simulink model "Tarea1"  (R2022a)
settings: Solver=VariableStepAuto  StartTime=0.0  StopTime=10.0  RelTol=1e-3
values from neighbouring files (symbols this model uses):
  den = [0 (L*J) (R*J+L*B) (R*B+Km*Ka)]    [CompensadordicretoVelocidadLGR.m]    (also in Grafica_FuncionDeTransferencia.m = [1 0,1486 0,04365]; PIDExperiment.m = str2num(get(handles.den,'string')); Raices.m = [1 12.02 0.1393]; Smulacro_Parcial_Final.m = [1 0 30 15])
  num = [0 (Km)]    [CompensadordicretoVelocidadLGR.m]    (also in Grafica_FuncionDeTransferencia.m = [0,2087 0,1993]; PIDExperiment.m = str2num(get(handles.num,'string')); Raices.m = [0.393 0.2155]; Smulacro_Parcial_Final.m = [1 2])
settings Model: Creator=juane  LastModifiedBy=juane

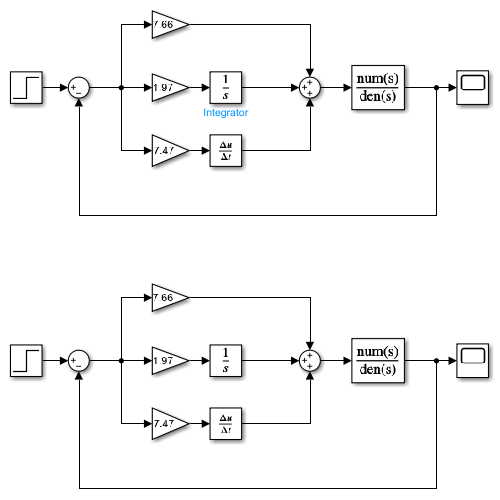
[thumbnail: Simulink's stored preview of the top-level diagram]
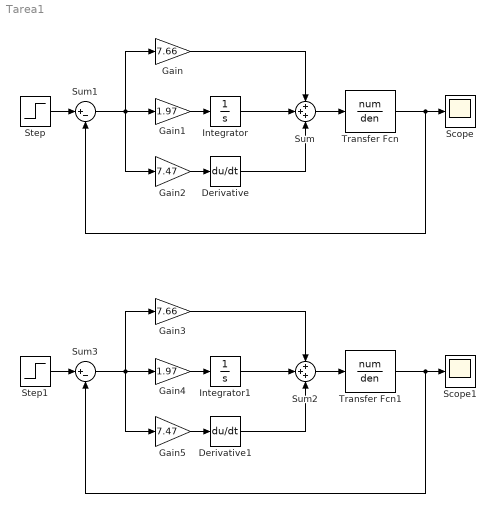
== system Tarea1 ==
  Derivative : Derivative
  Derivative1 : Derivative
  Gain : Gain  Gain=7.66
  Gain1 : Gain  Gain=1.97
  Gain2 : Gain  Gain=7.47
  Gain3 : Gain  Gain=7.66
  Gain4 : Gain  Gain=1.97
  Gain5 : Gain  Gain=7.47
  Integrator : Integrator
  Integrator1 : Integrator
  Scope : Scope
  Scope1 : Scope
  Step : Step  SampleTime=0
  Step1 : Step  SampleTime=0
  Sum : Sum  Inputs=+++
  Sum1 : Sum  Inputs=|+-
  Sum2 : Sum  Inputs=+++
  Sum3 : Sum  Inputs=|+-
  Transfer Fcn : TransferFcn  Numerator=num  Denominator=den
  Transfer Fcn1 : TransferFcn  Numerator=num  Denominator=den
  wires:
  Gain2/1 -> Derivative/1
  Gain1/1 -> Integrator/1
  Gain/1 -> Sum/1
  Integrator/1 -> Sum/2
  Derivative/1 -> Sum/3
  Sum/1 -> Transfer Fcn/1
  Transfer Fcn/1 -> Sum1/2, Scope/1
  Step/1 -> Sum1/1
  Sum1/1 -> Gain2/1, Gain1/1, Gain/1
  Transfer Fcn1/1 -> Sum3/2, Scope1/1
  Step1/1 -> Sum3/1
  Derivative1/1 -> Sum2/3
  Integrator1/1 -> Sum2/2
  Sum3/1 -> Gain5/1, Gain4/1, Gain3/1
  Sum2/1 -> Transfer Fcn1/1
  Gain4/1 -> Integrator1/1
  Gain5/1 -> Derivative1/1
  Gain3/1 -> Sum2/1
